simulink model "DC_Motor_Regulation"  (R2023b)
settings: Solver=VariableStepAuto  StartTime=0.0  StopTime=10  RelTol=1e-3
StopFcn:
  | show_results_after_sim
values from neighbouring files (symbols this model uses):
  Bm = 0.006126    [parameters.m]
  ke = 1.8    [parameters.m]
  kt = 1.8    [parameters.m]
  Ra = 0.1514    [parameters.m]
  Su = 9.5492    [parameters.m]
libraries: Lab_b x3, sps_lib x1
settings Model: Creator=Student  LastModifiedBy=Student
settings DataIOCC: LoggingFileName=logsout

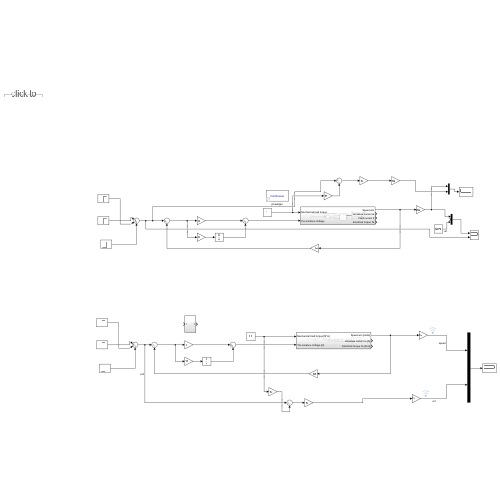
[thumbnail: Simulink's stored preview of the top-level diagram]
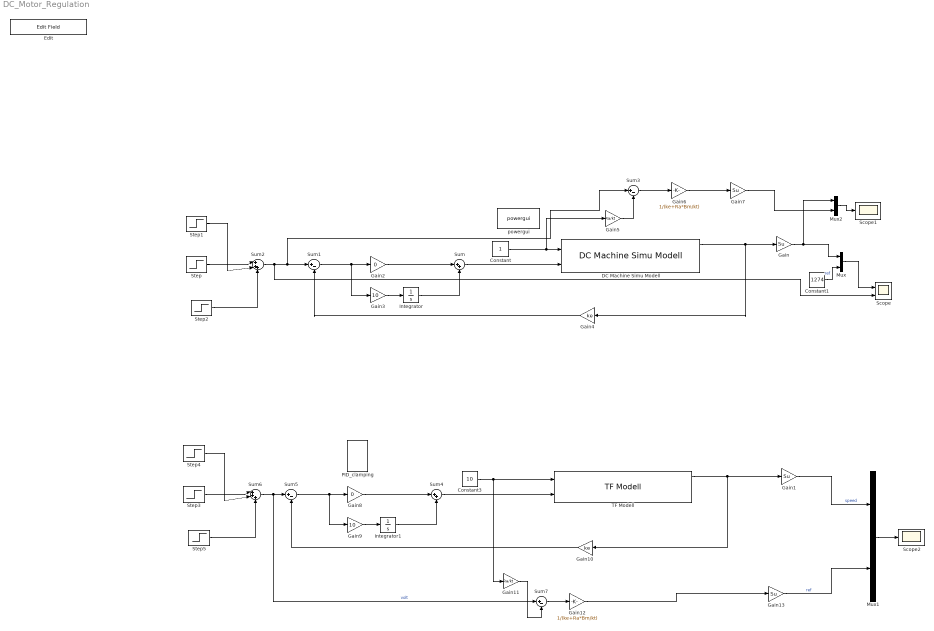
== system DC_Motor_Regulation ==
  Constant : Constant
  Constant1 : Constant  Value=1274
  Constant3 : Constant  Value=10
  DC Machine Simu Modell : Lab_b/DC Machine Simu Modell  SystemSampleTime=-1  VariantActivationTime=update diagram  AllowFlexibleInterface=on  Latency=0  AutoFrameSizeCalculation=off
  Edit : EditField  LabelPosition=Hide  ShowInitialText=on  Alignment=Center
  Gain{,1,7,13} (4 alike) : Gain  Gain=Su
  Gain10 : Gain  Gain=ke
  Gain11 : Gain  Gain=Ra/kt
  Gain12 : Gain  Gain=1/(ke+Ra*Bm/kt)
  Gain2 : Gain  Gain=0
  Gain3 : Gain  Gain=10
  Gain4 : Gain  Gain=ke
  Gain5 : Gain  Gain=Ra/kt
  Gain6 : Gain  Gain=1/(ke+Ra*Bm/kt)
  Gain8 : Gain  Gain=0
  Gain9 : Gain  Gain=10
  Integrator : Integrator
  Integrator1 : Integrator
  Mux : Mux  Inputs=3
  Mux1 : Mux  Inputs=2
  Mux2 : Mux  Inputs=2
  PID_clamping : Lab_b/PID_clamping  SystemSampleTime=-1  VariantActivationTime=update diagram  AllowFlexibleInterface=on  Latency=0  AutoFrameSizeCalculation=off
  Scope : Scope  NumInputPorts=2
  Scope1 : Scope
  Scope2 : Scope
  Step : Step  Time=5.5  After=50  SampleTime=0
  Step1 : Step  Time=8.2  After=50  SampleTime=0
  Step2 : Step  Time=1.1  After=200  SampleTime=0
  Step3 : Step  Time=5.5  After=50  SampleTime=0
  Step4 : Step  Time=8.2  After=150  SampleTime=0
  Step5 : Step  Time=1.1  After=80  SampleTime=0
  Sum : Sum  Inputs=|++
  Sum{1,3,5,7} (4 alike) : Sum  Inputs=|+-
  Sum2 : Sum  Inputs=|+++
  Sum4 : Sum  Inputs=|++
  Sum6 : Sum  Inputs=|+++
  TF Modell : Lab_b/TF Modell  SystemSampleTime=-1  VariantActivationTime=update diagram  AllowFlexibleInterface=on  Latency=0  AutoFrameSizeCalculation=off
      link override Transfer Fcn: Denominator=[La Ra]
  powergui : sps_lib/powergui  Priority=1  SimulationMode=Continuous  SampleTime=50e-6  frequency=60  Iterations=50  frequencyindice=0  Pbase=100e6  ErrMax=1e-4  UnitsV=kV  UnitsW=MW  buscounter=0  FunctionMessages=off  echomessages=off  EnableUseOfTLC=off  CurrentSourceSwitches=off  DisableSnubberDevices=off  DisableRonSwitches=off  DisableVfSwitches=off  DisplayEquations=off  AutomaticDiscreteSolvers=off  SolverType=Tustin/Backward Euler (TBE)  Interpol=off  ExternalGateDelay=off  methode=off  Ts=100  x0status=blocks  SPID=on  SwTol=0  HookPort=off  NonlinearTolerance=1e-4  nMaxIteration=100  ContinueOnMaxIteration=off  RestoreLinks=warning  ResistiveCurrentMeasurement=off  Frange=[0:2:500]  Ylog=off  Xlog=on  ShowGrid=off  save=off  variable=ZData  structure=0  ZoomFFT=off  StartTime=0.0  cycles=1  DisplayStyle=1  fundamental=60  FreqAxis=off  MaxFrequency=1000  frequencyindicesteady=1  RmsSteady=1  display=off
  wires:
  DC Machine Simu Modell/1 -> Gain4/1, Gain/1
  TF Modell/1 -> Gain10/1, Gain1/1
  Mux/1 -> Scope/1
  Gain/1 -> Mux2/1, Mux/1
  Constant1/1 -> Mux/3  "ref"
  Integrator/1 -> Sum/2
  Gain3/1 -> Integrator/1
  Gain2/1 -> Sum/1
  Sum1/1 -> Gain3/1, Gain2/1
  Sum/1 -> DC Machine Simu Modell/2
  Constant/1 -> Gain5/1, DC Machine Simu Modell/1
  Gain4/1 -> Sum1/2
  Step/1 -> Sum2/1
  Sum2/1 -> Scope/2, Sum3/1, Sum1/1
  Step1/1 -> Sum2/2
  Mux2/1 -> Scope1/1
  Gain5/1 -> Sum3/2
  Sum3/1 -> Gain6/1
  Gain6/1 -> Gain7/1
  Gain7/1 -> Mux2/2
  Step2/1 -> Sum2/3
  Gain1/1 -> Mux1/1  "speed"
  Sum5/1 -> Gain9/1, Gain8/1
  Gain8/1 -> Sum4/1
  Gain9/1 -> Integrator1/1
  Integrator1/1 -> Sum4/2
  Step5/1 -> Sum6/3
  Step4/1 -> Sum6/2
  Step3/1 -> Sum6/1
  Sum6/1 -> Sum7/1, Sum5/1  "volt"
  Gain13/1 -> Mux1/2  "ref"
  Gain12/1 -> Gain13/1
  Sum7/1 -> Gain12/1
  Gain11/1 -> Sum7/2
  Constant3/1 -> Gain11/1, TF Modell/1
  Mux1/1 -> Scope2/1
  Gain10/1 -> Sum5/2
  Sum4/1 -> TF Modell/2
